simulink library "lib_transmission2"  (Simulink 4.1.1)
values from neighbouring files (symbols this model uses):
  logFlag = 1    [advSACompMaskInit.m]    (also in advSACompMaskInitR13.m)
undefined symbols (not defined in the file or in its folder): cyc_mph, fc_map_spd, fc_max_trq, fc_spd_scale, fc_trq_scale, fd_inertia, fd_loss, fd_ratio, gb_dnshift_load, gb_dnshift_spd, gb_gear_number_lookup, gb_gears_num, gb_inertia, gb_loss_const, gb_loss_input_spd_coeff, gb_loss_input_trq_coeff, gb_loss_output_spd_coeff, gb_loss_output_trq_coeff, gb_map_spd_out, gb_map_trq_in, gb_map_trq_out, gb_num_init, gb_ratio, gb_shift_delay, gb_spd_scale, gb_trq_scale, gb_upshift_load, gb_upshift_spd, htc_inertia, htc_k_adv, htc_k_adv_coast, htc_lockup, htc_lockup_load, htc_lockup_spd, htc_lu_gear_range, htc_max_coast_tr, htc_min_coast_tr, htc_pump_loss_spd, htc_pump_loss_trq_lockup, htc_pump_loss_trq_unlock, htc_sr, htc_sr_coast, htc_tr, htc_tr_coast, htc_unlock_spd, mc_map_spd, mc_max_trq, mc_overtrq_factor, mc_spd_scale, mc_trq_scale, tc_loss, tc_mc_to_fc_ratio, tx_eff_map, tx_map_spd, tx_map_trq, tx_pg_r, tx_pg_s, tx_speed_dep, vc_clutch_bool, vc_idle_spd ... (+2)
libraries: lib_controls x1, lib_etc x1, lib_controls2 x1, lib_transmission x1
(part 1 of 17)
settings Model: LastModifiedBy=mokeefe
settings Model: ModifiedComment=|
  | tmarkel -- Fri Sep 20 16:05:52 2002 -- Version 1.102
  | modified Pout/Pin calc block - moved !=0 check to before bombproof block; value after bombproof is never zero
  | 
  | there are still some issues with this calculation to be resolved at a later date
settings Model: ModifiedHistory=|
  | tmarkel -- Fri Sep 20 16:05:52 2002 -- Version 1.102
  | modified Pout/Pin calc block - moved !=0 check to before bombproof block; value after bombproof is never zero
  | 
  | there are still some issues with this calculation to be resolved at a later date
  | 
  | 
  | tmarkel -- Fri Sep 20 16:05:52 2002 -- Version 1.102
  | modified Pout/Pin calc block - moved !=0 check to before bombproof block; value after bombproof is never zero
  | 
  | there are still some issues with this calculation to be resolved at a later date
  | 
  | 
  | tmarkel -- Fri Sep 20 14:16:55 2002 -- Version 1.101
  | changed t loss when tx_eff=0 to be the total torque in request
  | 
  | abrooker -- Fri May 24 14:07:33 2002 -- Version 1.100
  | 
  | mokeefe -- Thu Apr 18 08:38:43 2002 -- Version 1.99
  | saving the model:
  | o "without the model browser open"
  | o with only top-level screen visible
  | o with "fit to view" enabled
  | o with "status bar" off and "toolbar" off
  | o with "prompt to update model history with each save" on

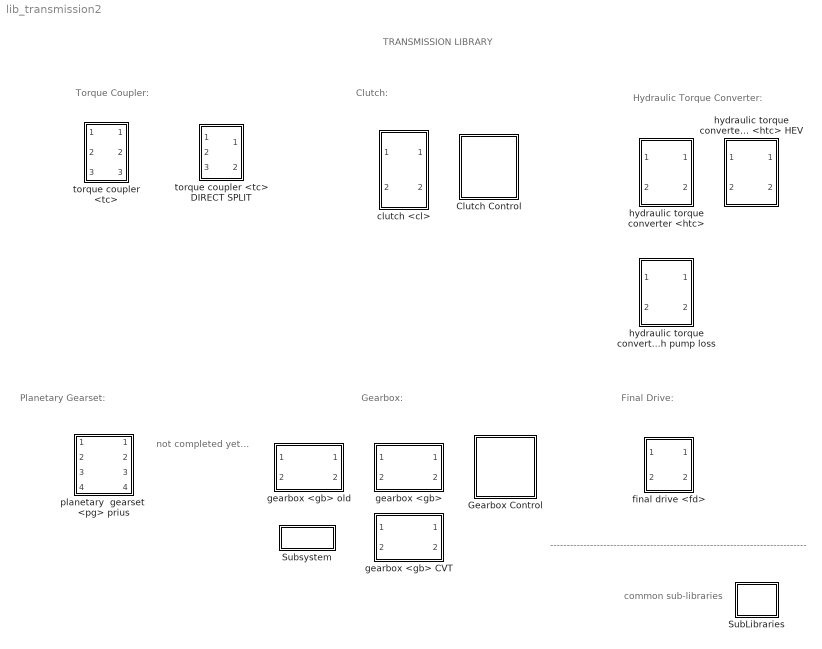
== system lib_transmission2 ==
  note: Torque Coupler:
  note: -----------------------------------------------------------------------------
  note: common
      | sub-libraries
  note: Clutch:
  note: Gearbox:
  note: Final Drive:
  note: Hydraulic Torque Converter:
  note: Planetary Gearset:
  note: not completed yet...
  note: TRANSMISSION LIBRARY
  Clutch Control : Subsystem
      settings: RTWFcnNameOpts=Auto  RTWFileNameOpts=Auto
  Gearbox Control : Subsystem
      settings: RTWFcnNameOpts=Auto  RTWFileNameOpts=Auto
  SubLibraries : Subsystem
      settings: RTWFcnNameOpts=Auto  RTWFileNameOpts=Auto
  Subsystem : Subsystem
      settings: RTWFcnNameOpts=Auto  RTWFileNameOpts=Auto
      mask Display: disp('GB Notes')
  clutch <cl> : Subsystem  mask(Stand-Alone Clutch Mask){generalName='cl', logPick=Don't Log, initFileName={}, modCell={}, imgFileName='bdi_cl.jpg', slip_spd=vc_launch_spd, maxtrq=max(fc_max_trq)*fc_trq_scale, DEBUG=OFF}
      mask prompts: generalName "General Name of this Component [char--evaluated]"; logPick "Log Variables to Workspace?"; initFileName "Initialization File(s) [cell array of char]"; modCell "Modification Cell [2 column cell array of param and val]"; imgFileName "Icon image file name [char--evaluated]"; slip_spd "Input shaft speed when clutch slips (rad/s):"; maxtrq "Maximum torque clutch can transmit:"
      mask help: Clutch for use with ADVISOR 2
      mask init:
      | % initialization via m-file script
      | advSACompMaskInit;
      settings: RTWFcnNameOpts=Auto  RTWFileNameOpts=Auto
      mask Help:
      | First input is req'd clutch output torque and speed, muxed together.
      | Second input is clutch state, with 1 => disengaged, 2 => slipping, and 3=> engaged.
      | Third input is available clutch input torque and limited clutch input speed.
      | First output is req'd clutch input torque and speed, muxed together.
      | Second output is available clutch output torque and limited clutch output speed.
      | The logic implemented by this block is as follows:
      |           IF (clutch is disengaged) THEN (req'd input torque=0), (req'd input speed=req'd output speed (the engine control is responsible for computing correct engine spin-down speed)), (avail. output torque=0), (limited output speed=req'd output speed)
      |           IF (clutch is slipping) THEN (req'd input torque=req'd output torque), (req'd input speed=user-defined slip speed), (avail. output torque=avail. input torque), (limited output speed=req'd output speed)
      |           IF (clutch is engaged) THEN (req'd input torque=req'd output torque), (req'd input speed=req'd output speed), (avail. output torque=avail. input torque), (limited output speed=limited input speed)
      | 
      | The clutch will transmit no more than its maximum torque as driving or braking torque.
      mask StyleString: edit,popup(Don't Log|Log),edit,edit,edit,edit,edit,popup(ON|OFF)
      mask Display: image(imread(imgFileName))
  final drive <fd> : Subsystem  mask(Stand-Alone Final Drive Mask){generalName='fd', logPick=Log, initFileName={}, modCell={}, imgFileName='bdi_fd.jpg', DEBUG=OFF}
      mask prompts: generalName "General Name of this Component [char]"; logPick "Log Variables to Workspace?"; initFileName "Initialization File(s) [cell array of char]"; modCell "Modification Cell [2 column cell array of param and val]"; imgFileName "Icon image file name [char--evaluated]"
      mask init:
      | % initialization via m-file script
      | advSACompMaskInit;
      settings: RTWFcnNameOpts=Auto  RTWFileNameOpts=Auto
      mask StyleString: edit,popup(Don't Log|Log),edit,edit,edit,popup(ON|OFF)
      mask Display: image(imread(imgFileName))
  gearbox <gb> : Subsystem  mask(Stand-Alone Gearbox Mask){generalName='gb', logPick=Log, initFileName={}, modCell={}, imgFileName='bdi_gb.jpg', DEBUG=OFF}
      mask prompts: generalName "General Name of this Component [char]"; logPick "Log Variables to Workspace?"; initFileName "Initialization File(s) [cell array of char]"; modCell "Modification Cell [2 column cell array of param and val]"; imgFileName "Icon image file name [char--evaluated]"
      mask init:
      | % initialization via m-file script
      | advSACompMaskInit;
      settings: RTWFcnNameOpts=Auto  RTWFileNameOpts=Auto
      mask StyleString: edit,popup(Don't Log|Log),edit,edit,edit,popup(ON|OFF)
      mask Display: image(imread(imgFileName))
  gearbox <gb> CVT : Subsystem  mask(Stand-Alone Gearbox Mask){generalName='gb', logPick=Log, initFileName={}, modCell={}, imgFileName='bdi_gb.jpg', DEBUG=OFF}
      mask prompts: generalName "General Name of this Component [char]"; logPick "Log Variables to Workspace?"; initFileName "Initialization File(s) [cell array of char]"; modCell "Modification Cell [2 column cell array of param and val]"; imgFileName "Icon image file name [char--evaluated]"
      mask init:
      | % initialization via m-file script
      | advSACompMaskInit;
      settings: RTWFcnNameOpts=Auto  RTWFileNameOpts=Auto
      mask StyleString: edit,popup(Don't Log|Log),edit,edit,edit,popup(ON|OFF)
      mask Display: image(imread(imgFileName))
  gearbox <gb> old : Subsystem  mask(Stand-Alone Gearbox Mask){generalName='gb', logPick=Log, initFileName={}, modCell={}, imgFileName='bdi_gb.jpg', DEBUG=OFF}
      mask prompts: generalName "General Name of this Component [char]"; logPick "Log Variables to Workspace?"; initFileName "Initialization File(s) [cell array of char]"; modCell "Modification Cell [2 column cell array of param and val]"; imgFileName "Icon image file name [char--evaluated]"
      mask init:
      | % initialization via m-file script
      | advSACompMaskInit;
      settings: RTWFcnNameOpts=Auto  RTWFileNameOpts=Auto
      mask StyleString: edit,popup(Don't Log|Log),edit,edit,edit,popup(ON|OFF)
      mask Display: image(imread(imgFileName))
  hydraulic torque converter <htc> : Subsystem  mask(Stand-Alone HTC Mask){generalName='htc', logPick=Log, initFileName={}, modCell={}, imgFileName='bdi_htc.jpg', DEBUG=OFF}
      mask prompts: generalName "General Name of this Component [char]"; logPick "Log Variables to Workspace?"; initFileName "Initialization File(s) [cell array of char]"; modCell "Modification Cell [2 column cell array of param and val]"; imgFileName "Icon image file name [char--evaluated]"
      mask init:
      | % initialization via m-file script
      | advSACompMaskInit;
      settings: RTWFcnNameOpts=Auto  RTWFileNameOpts=Auto
      mask StyleString: edit,popup(Don't Log|Log),edit,edit,edit,popup(ON|OFF)
      mask Display: image(imread(imgFileName))
  hydraulic torque converter <htc> HEV : Subsystem  mask(Stand-Alone HTC Mask){generalName='htc', logPick=Log, initFileName={}, modCell={}, imgFileName='bdi_htc.jpg', DEBUG=OFF}
      mask prompts: generalName "General Name of this Component [char]"; logPick "Log Variables to Workspace?"; initFileName "Initialization File(s) [cell array of char]"; modCell "Modification Cell [2 column cell array of param and val]"; imgFileName "Icon image file name [char--evaluated]"
      mask init:
      | % initialization via m-file script
      | advSACompMaskInit;
      settings: RTWFcnNameOpts=Auto  RTWFileNameOpts=Auto
      mask StyleString: edit,popup(Don't Log|Log),edit,edit,edit,popup(ON|OFF)
      mask Display: image(imread(imgFileName))
  hydraulic torque converter <htc> with pump loss : Subsystem  mask(Stand-Alone HTC Mask){generalName='htc', logPick=Log, initFileName={}, modCell={}, imgFileName='bdi_htc.jpg', DEBUG=OFF}
      mask prompts: generalName "General Name of this Component [char]"; logPick "Log Variables to Workspace?"; initFileName "Initialization File(s) [cell array of char]"; modCell "Modification Cell [2 column cell array of param and val]"; imgFileName "Icon image file name [char--evaluated]"
      mask init:
      | % initialization via m-file script
      | advSACompMaskInit;
      settings: RTWFcnNameOpts=Auto  RTWFileNameOpts=Auto
      mask StyleString: edit,popup(Don't Log|Log),edit,edit,edit,popup(ON|OFF)
      mask Display: image(imread(imgFileName))
  planetary  gearset  <pg> prius : Subsystem
      settings: RTWFcnNameOpts=Auto  RTWFileNameOpts=Auto
      mask Display: image(imread('bdi_psplit.jpg'))
  torque coupler <tc> : Subsystem  mask(Stand-Alone Torque Coupler Mask){generalName='tc', logPick=Don't Log, initFileName={}, modCell={}, imgFileName='bdi_tc.jpg', DEBUG=OFF}
      mask prompts: generalName "General Name of this Component [char--evaluated]"; logPick "Log Variables to Workspace?"; initFileName "Initialization File(s) [cell array of char]"; modCell "Modification Cell [2 column cell array of param and val]"; imgFileName "Icon image file name [char--evaluated]"
      mask init:
      | % initialization via m-file script
      | advSACompMaskInit;
      settings: RTWFcnNameOpts=Auto  RTWFileNameOpts=Auto
      mask StyleString: edit,popup(Don't Log|Log),edit,edit,edit,popup(ON|OFF)
      mask Display: image(imread(imgFileName))
  torque coupler <tc> DIRECT SPLIT : Subsystem  mask(Stand-Alone Direct Split Torque Coupler Mask){generalName='tc', logPick=Log, initFileName={}, modCell={}, imgFileName='bdi_tc.jpg', DEBUG=OFF}
      mask prompts: generalName "General Name of this Component [char--evaluated]"; logPick "Log Variables to Workspace?"; initFileName "Initialization File(s) [cell array of char]"; modCell "Modification Cell [2 column cell array of param and val]"; imgFileName "Icon image file name [char--evaluated]"
      mask init:
      | % initialization via m-file script
      | advSACompMaskInit;
      settings: RTWFcnNameOpts=Auto  RTWFileNameOpts=Auto
      mask StyleString: edit,popup(Don't Log|Log),edit,edit,edit,popup(ON|OFF)
      mask Display: image(imread(imgFileName))

== system lib_transmission2/Clutch Control ==
  Clutch Control : Subsystem
      settings: RTWFcnNameOpts=Auto  RTWFileNameOpts=Auto

== system lib_transmission2/Gearbox Control ==
  Gearbox Control manual shift logic : Subsystem
      settings: RTWFcnNameOpts=Auto  RTWFileNameOpts=Auto
  automatic transmission gearbox and htc advanced lock-up logic for htc shift logic for gearbox : Subsystem
      settings: RTWFcnNameOpts=Auto  RTWFileNameOpts=Auto
  automatic transmission gearbox and htc standard lockup logic for htc shift logic for gearbox : Subsystem
      settings: RTWFcnNameOpts=Auto  RTWFileNameOpts=Auto
  time lookup shift logic for gearbox : Subsystem
      settings: RTWFcnNameOpts=Auto  RTWFileNameOpts=Auto
  vehicle speed dependent shift logic for gearbox : Subsystem
      settings: RTWFcnNameOpts=Auto  RTWFileNameOpts=Auto

== system lib_transmission2/SubLibraries ==
  note: Trq and Spd at Output
      | (Nm) and (rad/s)
  note: Gear Ratio
      | (input spd/output spd)
  note: Trq loss
      | at input (Nm)
  note: gear ratio
      | (input/output spd)
  note: gear (1st, 2nd, etc.)
  note: data needs:
      | gb_ratio
  note: Below is the loss block for a gear box based
      | on loss equation--used with ADVISOR v. 3.1 and below
  note: X_lookup
  note: Y_lookup
  note: Z_discrete value
  note: looked up value
  note: X_lookup
  note: Y_lookup
  note: Z_discrete value
  note: looked up value
  3D discrete lookup table : Subsystem  mask{tx_map_spd=tx_map_spd, tx_map_trq=tx_map_trq, tx_eff_map=tx_eff_map}
      mask prompts: tx_map_spd "Row Lookup"; tx_map_trq "Column Lookup"; tx_eff_map "Lookup Matrix"
      settings: RTWFcnNameOpts=Auto  RTWFileNameOpts=Auto
  3D discrete lookup table (sfun) : Subsystem  mask{tx_map_spd=tx_map_spd, tx_map_trq=tx_map_trq, tx_eff_map=tx_eff_map}
      mask prompts: tx_map_spd "Row Lookup"; tx_map_trq "Column Lookup"; tx_eff_map "Lookup Matrix"
      settings: RTWFcnNameOpts=Auto  RTWFileNameOpts=Auto
  "gear determination (e.g., 1st gear, 2nd, etc.)" : Subsystem
      settings: RTWFcnNameOpts=Auto  RTWFileNameOpts=Auto
  loss (Nm) : Subsystem  mask{tx_eff_map=tx_eff_map, tx_map_trq=tx_map_trq, tx_map_spd=tx_map_spd, gb_spd_scale=gb_spd_scale, gb_trq_scale=gb_trq_scale}
      mask prompts: tx_eff_map "table of efficiency values (spd rad/s, trq Nm)"; tx_map_trq "vector of output torque values for lookup table (Nm)"; tx_map_spd "vector of output speeds for lookup table (rad/s)"; gb_spd_scale "Speed scale for the transmission gear box"; gb_trq_scale "Torque scale for the transmission gear box"
      settings: RTWFcnNameOpts=Auto  RTWFileNameOpts=Auto
  loss (Nm) old methodology : Subsystem
      settings: RTWFcnNameOpts=Auto  RTWFileNameOpts=Auto
  notes on  3D discrete lookup table : Subsystem
      settings: RTWFcnNameOpts=Auto  RTWFileNameOpts=Auto
  notes on  loss (Nm) : Subsystem
      settings: RTWFcnNameOpts=Auto  RTWFileNameOpts=Auto

== system lib_transmission2/Subsystem ==
  note: The gearbox old
      | model uses transmission
      | efficiency referenced from
      | the transmission output.
      |
      | The new file references from
      | the input.

== system lib_transmission2/clutch <cl> ==
  note: Clutch
      | Interface
  T & w output requested : Inport  Port=1  LatchInput=off
  T & w input achieved : Inport  Port=2  LatchInput=off
  clutch model and interface : Subsystem
      settings: RTWFcnNameOpts=Auto  RTWFileNameOpts=Auto
  T & w input request : Outport  Port=1
  T & w output achieved : Outport  Port=2
  tag scope: clReqOut=global, clSensors=global
  wires:
  T & w output requested/1 -> clutch model and interface/1(T & w output requested)
  clutch model and interface/2(Out1) -> T & w input request/1
  T & w input achieved/1 -> clutch model and interface/2(T & w input achieved)
  clutch model and interface/3(Out2) -> T & w output achieved/1
  clutch model and interface/4(sensors) -> [clSensors]
  clutch model and interface/1(required out) -> [clReqOut]
  [clControl] -> clutch model and interface/3(control)

== system lib_transmission2/final drive <fd> ==
  "torque and speed req'd at output side of final drive (Nm), (rad/s)" : Inport  Port=1  LatchInput=off
  "torque and speed avail. at input side of final drive (Nm), (rad/s)" : Inport  Port=2  LatchInput=off
  Block NOTES : Subsystem
      settings: RTWFcnNameOpts=Auto  RTWFileNameOpts=Auto
      mask Display: disp('Block\nNOTES')
  help : Subsystem
      settings: OpenFcn=web(['file:\\\' which('wheel_axle.htm')]);  RTWFcnNameOpts=Auto  RTWFileNameOpts=Auto
      mask Display: image(imread('doc_man.jpg'))
  model&interface : Subsystem
      settings: RTWFcnNameOpts=Auto  RTWFileNameOpts=Auto
  "torque and speed req'd at input side of final drive (Nm), (rad/s)" : Outport  Port=1  InitialOutput=0
  "torque and speed avail. at output side of final drive (Nm), (rad/s)" : Outport  Port=2  InitialOutput=0
  tag scope: fdReqOut=global, fdSensors=global
  wires:
  model&interface/1(out request) -> [fdReqOut]
  [fdControl] -> model&interface/3(control)
  model&interface/4(sensors) -> [fdSensors]
  "torque and speed req'd at output side of final drive (Nm), (rad/s)"/1 -> model&interface/1(T & w output request)
  "torque and speed avail. at input side of final drive (Nm), (rad/s)"/1 -> model&interface/2(T & w input achieved)
  model&interface/2(T & w input request) -> "torque and speed req'd at input side of final drive (Nm), (rad/s)"/1
  model&interface/3(T & w output achieved) -> "torque and speed avail. at output side of final drive (Nm), (rad/s)"/1

== system lib_transmission2/gearbox <gb> ==
  note: Gearbox
  "torque and speed req'd at output side of gearbox (Nm), (rad/s)" : Inport  Port=1  LatchInput=off
  "torque and speed avail. at input side of gearbox (Nm), (rad/s)" : Inport  Port=2  LatchInput=off
  Block NOTES : Subsystem
      settings: RTWFcnNameOpts=Auto  RTWFileNameOpts=Auto
      mask Display: disp('Block\nNOTES')
  gearbox model & interface : Subsystem
      settings: RTWFcnNameOpts=Auto  RTWFileNameOpts=Auto
  help : Subsystem
      settings: OpenFcn=web(['file:\\\' which('gearbox.htm')]);  RTWFcnNameOpts=Auto  RTWFileNameOpts=Auto
      mask Display: image(imread('doc_man.jpg'))
  "torque and speed req'd at input side of gearbox (Nm), (rad/s)" : Outport  Port=1  InitialOutput=0
  "torque and speed avail. at output side of gearbox (Nm), (rad/s)" : Outport  Port=2  InitialOutput=0
  tag scope: gbReqOut=global, gbSensors=global
  wires:
  gearbox model & interface/1(requested output) -> [gbReqOut]
  gearbox model & interface/2(trq and spd input request) -> "torque and speed req'd at input side of gearbox (Nm), (rad/s)"/1
  "torque and speed req'd at output side of gearbox (Nm), (rad/s)"/1 -> gearbox model & interface/1(trq and spd output request)
  "torque and speed avail. at input side of gearbox (Nm), (rad/s)"/1 -> gearbox model & interface/2(trq and spd input achieved)
  gearbox model & interface/3(trq and spd output achieved) -> "torque and speed avail. at output side of gearbox (Nm), (rad/s)"/1
  [gbControl] -> gearbox model & interface/3(controls)
  gearbox model & interface/4(sensors) -> [gbSensors]

== system lib_transmission2/gearbox <gb> CVT ==
  note: Gearbox
  "torque and speed req'd at output side of gearbox (Nm), (rad/s)" : Inport  Port=1  LatchInput=off
  "torque and speed avail. at input side of gearbox (Nm), (rad/s)" : Inport  Port=2  LatchInput=off
  Block NOTES : Subsystem
      settings: RTWFcnNameOpts=Auto  RTWFileNameOpts=Auto
      mask Display: disp('Block\nNOTES')
  CVT model & interface : Subsystem
      settings: RTWFcnNameOpts=Auto  RTWFileNameOpts=Auto
  help : Subsystem
      settings: OpenFcn=web(['file:\\\' which('gearbox.htm')]);  RTWFcnNameOpts=Auto  RTWFileNameOpts=Auto
      mask Display: image(imread('doc_man.jpg'))
  "torque and speed req'd at input side of gearbox (Nm), (rad/s)" : Outport  Port=1  InitialOutput=0
  "torque and speed avail. at output side of gearbox (Nm), (rad/s)" : Outport  Port=2  InitialOutput=0
  tag scope: gbReqOut=global, gbSensors=global
  wires:
  CVT model & interface/1(requested output) -> [gbReqOut]
  CVT model & interface/2(trq and spd input request) -> "torque and speed req'd at input side of gearbox (Nm), (rad/s)"/1
  "torque and speed req'd at output side of gearbox (Nm), (rad/s)"/1 -> CVT model & interface/1(trq and spd output request)
  "torque and speed avail. at input side of gearbox (Nm), (rad/s)"/1 -> CVT model & interface/2(trq and spd input achieved)
  CVT model & interface/3(trq and spd output achieved) -> "torque and speed avail. at output side of gearbox (Nm), (rad/s)"/1
  [gbControl] -> CVT model & interface/3(controls)
  CVT model & interface/4(sensors) -> [gbSensors]

== system lib_transmission2/gearbox <gb> old ==
  note: Gearbox
  "torque and speed req'd at output side of gearbox (Nm), (rad/s)" : Inport  Port=1  LatchInput=off
  "torque and speed avail. at input side of gearbox (Nm), (rad/s)" : Inport  Port=2  LatchInput=off
  Block NOTES : Subsystem
      settings: RTWFcnNameOpts=Auto  RTWFileNameOpts=Auto
      mask Display: disp('Block\nNOTES')
  gearbox model & interface : Subsystem
      settings: RTWFcnNameOpts=Auto  RTWFileNameOpts=Auto
  help : Subsystem
      settings: OpenFcn=web(['file:\\\' which('gearbox.htm')]);  RTWFcnNameOpts=Auto  RTWFileNameOpts=Auto
      mask Display: image(imread('doc_man.jpg'))
  "torque and speed req'd at input side of gearbox (Nm), (rad/s)" : Outport  Port=1  InitialOutput=0
  "torque and speed avail. at output side of gearbox (Nm), (rad/s)" : Outport  Port=2  InitialOutput=0
  tag scope: gbReqOut=global, gbSensors=global
  wires:
  gearbox model & interface/1(requested output) -> [gbReqOut]
  gearbox model & interface/2(trq and spd input request) -> "torque and speed req'd at input side of gearbox (Nm), (rad/s)"/1
  "torque and speed req'd at output side of gearbox (Nm), (rad/s)"/1 -> gearbox model & interface/1(trq and spd output request)
  "torque and speed avail. at input side of gearbox (Nm), (rad/s)"/1 -> gearbox model & interface/2(trq and spd input achieved)
  gearbox model & interface/3(trq and spd output achieved) -> "torque and speed avail. at output side of gearbox (Nm), (rad/s)"/1
  [gbControl] -> gearbox model & interface/3(controls)
  gearbox model & interface/4(sensors) -> [gbSensors]

== system lib_transmission2/hydraulic torque converter <htc> ==
  note: Hydraulic Torque Converter
  T & w output requested : Inport  Port=1  LatchInput=off
  T & w input available : Inport  Port=2  LatchInput=off
  conventional HTC  and Interface : Subsystem
      settings: RTWFcnNameOpts=Auto  RTWFileNameOpts=Auto
  T & w input requested : Outport  Port=1  InitialOutput=0
  T & w output available : Outport  Port=2  InitialOutput=0
  tag scope: htcReqOut=global, htcSensors=global
  wires:
  conventional HTC  and Interface/1(requested output) -> [htcReqOut]
  conventional HTC  and Interface/4(sensors) -> [htcSensors]
  conventional HTC  and Interface/2(trq and spd input request) -> T & w input requested/1
  conventional HTC  and Interface/3(trq and spd output achieved) -> T & w output available/1
  T & w output requested/1 -> conventional HTC  and Interface/1(trq and spd output request)
  T & w input available/1 -> conventional HTC  and Interface/2(trq and spd input achieved)
  [htcControl] -> conventional HTC  and Interface/3(control)

== system lib_transmission2/hydraulic torque converter <htc> HEV ==
  note: Hydraulic Torque Converter
  T & w output requested : Inport  Port=1  LatchInput=off
  T & w input available : Inport  Port=2  LatchInput=off
  HTC for parallel HEV and Interface : Subsystem
      settings: RTWFcnNameOpts=Auto  RTWFileNameOpts=Auto
  T & w input requested : Outport  Port=1  InitialOutput=0
  T & w output available : Outport  Port=2  InitialOutput=0
  tag scope: htcReqOut=global, htcSensors=global
  wires:
  HTC for parallel HEV and Interface/1(requested output) -> [htcReqOut]
  HTC for parallel HEV and Interface/4(sensors) -> [htcSensors]
  HTC for parallel HEV and Interface/2(trq and spd input request) -> T & w input requested/1
  HTC for parallel HEV and Interface/3(trq and spd output achieved) -> T & w output available/1
  T & w output requested/1 -> HTC for parallel HEV and Interface/1(trq and spd output request)
  T & w input available/1 -> HTC for parallel HEV and Interface/2(trq and spd input achieved)
  [htcControl] -> HTC for parallel HEV and Interface/3(control)

== system lib_transmission2/hydraulic torque converter <htc> with pump loss ==
  note: Hydraulic Torque Converter
  T & w output requested : Inport  Port=1  LatchInput=off
  T & w input available : Inport  Port=2  LatchInput=off
  conventional HTC  and Interface : Subsystem
      settings: RTWFcnNameOpts=Auto  RTWFileNameOpts=Auto
  T & w input requested : Outport  Port=1  InitialOutput=0
  T & w output available : Outport  Port=2  InitialOutput=0
  tag scope: htcReqOut=global, htcSensors=global
  wires:
  conventional HTC  and Interface/1(requested output) -> [htcReqOut]
  conventional HTC  and Interface/4(sensors) -> [htcSensors]
  conventional HTC  and Interface/2(trq and spd input request) -> T & w input requested/1
  conventional HTC  and Interface/3(trq and spd output achieved) -> T & w output available/1
  T & w output requested/1 -> conventional HTC  and Interface/1(trq and spd output request)
  T & w input available/1 -> conventional HTC  and Interface/2(trq and spd input achieved)
  [htcControl] -> conventional HTC  and Interface/3(control)

== system lib_transmission2/planetary  gearset  <pg> prius ==
  "torque and speed required from ring gear (Nm), (rad/s)1" : Inport  Port=1  LatchInput=off
  "torque and speed avail. from fuel converter (Nm), (rad/s)" : Inport  Port=2  LatchInput=off
  "torque and speed avail. from generator (Nm), (rad/s)" : Inport  Port=3  LatchInput=off
  "torque and speed available from motor (Nm), (rad/s)1" : Inport  Port=4  LatchInput=off
  Demux{,1..3} (4 alike) : Demux  Outputs=2  BusSelectionMode=off
  Mux{,1..3} (4 alike) : Mux  Inputs=2
      settings: DisplayOption=none
  Sum2 : Sum  Inputs=++  SaturateOnIntegerOverflow=on
  Sum5 : Sum  Inputs=+-  SaturateOnIntegerOverflow=on
  Sum6 : Sum  Inputs=+-  SaturateOnIntegerOverflow=on
  Terminator : Terminator
  Terminator2 : Terminator
  engine_to_generator : Gain  Gain=-tx_pg_s/(tx_pg_r+tx_pg_s)  Multiplication=Element-wise(K.*u)  SaturateOnIntegerOverflow=on
  gain : Gain  Gain=tx_pg_r/(tx_pg_r+tx_pg_s)  Multiplication=Element-wise(K.*u)  SaturateOnIntegerOverflow=on
  gain2 : Gain  Gain=1+tx_pg_r/tx_pg_s  Multiplication=Element-wise(K.*u)  SaturateOnIntegerOverflow=on
  gain5 : Gain  Gain=tx_pg_r/tx_pg_s  Multiplication=Element-wise(K.*u)  SaturateOnIntegerOverflow=on
  spd out : ToWorkspace  VariableName=pg_spd_out_r  SampleTime=0  SaveFormat=Array
      settings: MaxDataPoints=100000
  trq out : ToWorkspace  VariableName=pg_trq_out_r  SampleTime=0  SaveFormat=Array
      settings: MaxDataPoints=100000
  "torque and speed req'd from fuel converter (Nm), (rad/s)" : Outport  Port=1  InitialOutput=0
  "torque and speed req'd from generator (Nm), (rad/s)" : Outport  Port=2  InitialOutput=0
  "torque and speed req'd from motor (Nm), (rad/s)1" : Outport  Port=3  InitialOutput=0
  "torque and speed available to final drive (Nm), (rad/s)1" : Outport  Port=4  InitialOutput=0
  tag scope: pgs_trq_spd_r=global
  wires:
  "torque and speed available from motor (Nm), (rad/s)1"/1 -> Demux3/1
  Demux3/2 -> gain5/1, Mux3/2
  Demux3/1 -> Sum2/2
  Mux3/1 -> "torque and speed available to final drive (Nm), (rad/s)1"/1
  Sum2/1 -> Mux3/1
  Sum5/1 -> Mux1/2
  engine_to_generator/1 -> Mux1/1
  Mux1/1 -> "torque and speed req'd from generator (Nm), (rad/s)"/1
  Sum6/1 -> Mux2/1
  Mux2/1 -> "torque and speed req'd from motor (Nm), (rad/s)1"/1
  gain2/1 -> Sum5/1
  Demux/2 -> Terminator/1
  Demux/1 -> Terminator2/1
  "torque and speed avail. from generator (Nm), (rad/s)"/1 -> Demux/1
  Demux1/1 -> engine_to_generator/1, gain/1
  Demux1/2 -> gain2/1
  "torque and speed avail. from fuel converter (Nm), (rad/s)"/1 -> Demux1/1
  gain5/1 -> Sum5/2
  [fc_trq_req] -> Mux/1
  [fc_spd_req] -> Mux/2
  Mux/1 -> "torque and speed req'd from fuel converter (Nm), (rad/s)"/1
  Demux2/1 -> Sum6/1, trq out/1
  Demux2/2 -> Mux2/2, spd out/1
  gain/1 -> Sum2/1, Sum6/2
  "torque and speed required from ring gear (Nm), (rad/s)1"/1 -> [pgs_trq_spd_r], Demux2/1

== system lib_transmission2/torque coupler <tc> ==
  note: Torque Coupler
  "torque and speed req'd at output side of torque coupler (Nm), (rad/s)" : Inport  Port=1  LatchInput=off
  "torque and speed avail. at main input (Nm), (rad/s)" : Inport  Port=2  LatchInput=off
  "torque and speed avail. at motor input to tc (Nm), (rad/s)" : Inport  Port=3  LatchInput=off
  tc model & interface : Subsystem
      settings: RTWFcnNameOpts=Auto  RTWFileNameOpts=Auto
  "torque and speed req'd at main input to torque coupler (Nm), (rad/s)" : Outport  Port=1  InitialOutput=0
  "torque and speed req'd at motor input to torque coupler (Nm), (rad/s)" : Outport  Port=2  InitialOutput=0
  "torque and speed avail. at output side of torque coupler (Nm), (rad/s)" : Outport  Port=3  InitialOutput=0
  tag scope: tcReqOut=global, tcSensors=global
  wires:
  "torque and speed req'd at output side of torque coupler (Nm), (rad/s)"/1 -> tc model & interface/1(trq and spd output request)
  "torque and speed avail. at main input (Nm), (rad/s)"/1 -> tc model & interface/2(trq and spd avail. at main input)
  "torque and speed avail. at motor input to tc (Nm), (rad/s)"/1 -> tc model & interface/3(trq and spd avail. at motor input to tc)
  [tcControl] -> tc model & interface/4(controls)
  tc model & interface/1(requested output) -> [tcReqOut]
  tc model & interface/2(trq and spd req'd at main input) -> "torque and speed req'd at main input to torque coupler (Nm), (rad/s)"/1
  tc model & interface/3(trq and spd req'd at motor input to torque coupler) -> "torque and speed req'd at motor input to torque coupler (Nm), (rad/s)"/1
  tc model & interface/4(trq and spd avail. at output side of torque coupler) -> "torque and speed avail. at output side of torque coupler (Nm), (rad/s)"/1
  tc model & interface/5(sensors) -> [tcSensors]

== system lib_transmission2/torque coupler <tc> DIRECT SPLIT ==
  note: Torque Coupler
  "torque and speed req'd at output side of torque coupler (Nm), (rad/s)" : Inport  Port=1  LatchInput=off
  "torque and speed avail. at main input (Nm), (rad/s)" : Inport  Port=2  LatchInput=off
  "torque and speed avail. at motor input to tc (Nm), (rad/s)" : Inport  Port=3  LatchInput=off
  tc direct split model & interface : Subsystem
      settings: RTWFcnNameOpts=Auto  RTWFileNameOpts=Auto
  "torque and speed req'd at main input to torque coupler (Nm), (rad/s)" : Outport  Port=1  InitialOutput=0
  "torque and speed avail. at output side of torque coupler (Nm), (rad/s)" : Outport  Port=2  InitialOutput=0
  tag scope: tcReqOut=global, tcSensors=global
  wires:
  "torque and speed req'd at output side of torque coupler (Nm), (rad/s)"/1 -> tc direct split model & interface/1(trq and spd output request)
  "torque and speed avail. at main input (Nm), (rad/s)"/1 -> tc direct split model & interface/2(trq and spd avail. at main input)
  "torque and speed avail. at motor input to tc (Nm), (rad/s)"/1 -> tc direct split model & interface/3(trq and spd avail. at motor input to tc)
  [tcControl] -> tc direct split model & interface/4(control)
  tc direct split model & interface/1(required output) -> [tcReqOut]
  tc direct split model & interface/2(trq and spd req'd at main input) -> "torque and speed req'd at main input to torque coupler (Nm), (rad/s)"/1
  tc direct split model & interface/3(trq and spd avail. at output side of torque coupler) -> "torque and speed avail. at output side of torque coupler (Nm), (rad/s)"/1
  tc direct split model & interface/4(sensors) -> [tcSensors]

== system lib_transmission2/Clutch Control/Clutch Control ==
  Bus Creator : BusCreator  Inputs=3
  Bus Selector : BusSelector  OutputSignals=mpha  MuxedOutput=off
  Bus Selector1 : BusSelector  OutputSignals=shifting  MuxedOutput=off
  Bus Selector2 : BusSelector  OutputSignals=gb_spd_in_a  MuxedOutput=off
  Bus Selector3 : BusSelector  OutputSignals=clutch_trq_out_r  MuxedOutput=off
  Bus Selector4 : BusSelector  OutputSignals=clutch_spd_out_r  MuxedOutput=off
  Bus Selector5 : BusSelector  OutputSignals=veh_spd_a_rec  MuxedOutput=off
  Bus Selector6 : BusSelector  OutputSignals=cycle_mph_r  MuxedOutput=off
  Bus Selector7 : BusSelector  OutputSignals=v_ave_req  MuxedOutput=off
  Clutch Control : Subsystem  TreatAsAtomicUnit=on
      settings: RTWFcnNameOpts=Auto  RTWFileNameOpts=Auto
  Memory1 : Memory  X0=0  InheritSampleTime=off
      settings: RTWStateStorageClass=Auto
  Memory2 : Memory  X0=cyc_mph(1,2)  InheritSampleTime=off
      settings: RTWStateStorageClass=Auto
  Memory3 : Memory  X0=0  InheritSampleTime=off
      settings: RTWStateStorageClass=Auto
  Memory4 : Memory  X0=cyc_mph(1,2)  InheritSampleTime=off
      settings: RTWStateStorageClass=Auto
  tag scope: clControl=global
  wires:
  Memory4/1 -> Clutch Control/7(cyc_mph_r)
  Memory3/1 -> Clutch Control/6(veh_spd_a_rec)
  Memory2/1 -> Clutch Control/5(mpha)
  Memory1/1 -> Clutch Control/2(gb_spd_in_a)
  Clutch Control/3(launch_flag) -> Bus Creator/3  "launch_flag"
  Bus Selector4/1 -> Clutch Control/4(w_cl_out)  "<clutch_spd_out_r>"
  Bus Selector3/1 -> Clutch Control/3(T_cl_out)  "<clutch_trq_out_r>"
  [clReqOut] -> Bus Selector4/1, Bus Selector3/1
  Bus Selector2/1 -> Memory1/1  "<gb_spd_in_a>"
  [gbSensors] -> Bus Selector2/1
  Bus Selector1/1 -> Clutch Control/1(shifting)  "<shifting>"
  [gbControl] -> Bus Selector1/1
  Clutch Control/2(launch_speed) -> Bus Creator/2  "launch_speed"
  Clutch Control/1(clutch_state) -> Bus Creator/1  "clutch_state"
  Bus Creator/1 -> [clControl]
  [vehSensors] -> Bus Selector/1
  Bus Selector/1 -> Memory2/1  "<mpha>"
  [vehSensors] -> Bus Selector5/1
  Bus Selector5/1 -> Memory3/1  "<veh_spd_a_rec>"
  [cycReqOut] -> Bus Selector6/1
  Bus Selector6/1 -> Memory4/1  "<cycle_mph_r>"
  [vehReqOut] -> Bus Selector7/1
  Bus Selector7/1 -> Clutch Control/8(v_ave_req)  "<v_ave_req>"

== system lib_transmission2/Gearbox Control/Gearbox Control manual shift logic ==
  Bus Selector : BusSelector  OutputSignals=acc_mech_trq_a  MuxedOutput=off
  Bus Selector1 : BusSelector  OutputSignals=mpha  MuxedOutput=off
  Bus Selector10 : BusSelector  OutputSignals=eta_gb  MuxedOutput=off
  Bus Selector2 : BusSelector  OutputSignals=cycle_mph_r  MuxedOutput=off
  Bus Selector3 : BusSelector  OutputSignals=veh_spd_a_rec  MuxedOutput=off
  Bus Selector4 : BusSelector  OutputSignals=slip_limited  MuxedOutput=off
  Bus Selector7 : BusSelector  OutputSignals=gb_trq_out_r  MuxedOutput=off
  Bus Selector8 : BusSelector  OutputSignals=gb_spd_out_r  MuxedOutput=off
  Bus Selector9 : BusSelector  OutputSignals=gb_spd_in_a  MuxedOutput=off
  Memory{,1,3,5} (4 alike) : Memory  X0=0  InheritSampleTime=off
      settings: RTWStateStorageClass=Auto
  Memory2 : Memory  X0=cyc_mph(1,2)  InheritSampleTime=off
      settings: RTWStateStorageClass=Auto
  Memory4 : Memory  X0=cyc_mph(1,2)  InheritSampleTime=off
      settings: RTWStateStorageClass=Auto
  Mux1 : Mux  Inputs=3
  manual shift logic : Subsystem  TreatAsAtomicUnit=on
      settings: RTWFcnNameOpts=Auto  RTWFileNameOpts=Auto
  tag scope: gbControl=global
  wires:
  Memory4/1 -> manual shift logic/7("cyc_mph_r, t=(i-1)")
  Memory3/1 -> manual shift logic/8("veh_spd_a_rec, t=(i-1)")
  Memory2/1 -> manual shift logic/6("mpha, t=(i-1)")
  Memory1/1 -> manual shift logic/2("gb_spd_in_a, t=(i-1)")
  Memory/1 -> manual shift logic/1("eta_gb, t=(i-1)")
  [gbReqOut] -> Bus Selector7/1, Bus Selector8/1
  Bus Selector7/1 -> manual shift logic/4(T_gb_out)  "<gb_trq_out_r>"
  Bus Selector8/1 -> manual shift logic/3(w_gb_out)  "<gb_spd_out_r>"
  Bus Selector9/1 -> Memory1/1  "<gb_spd_in_a>"
  Bus Selector10/1 -> Memory/1  "<eta_gb>"
  [gbSensors] -> Bus Selector9/1, Bus Selector10/1
  Mux1/1 -> [gbControl]
  manual shift logic/3(gear number) -> Mux1/3  "gear_number"
  manual shift logic/2(shifting) -> Mux1/2  "shifting"
  manual shift logic/1(gear ratio) -> Mux1/1  "gear_ratio"
  [accSensors] -> Bus Selector/1
  Bus Selector/1 -> Memory5/1  "<acc_mech_trq_a>"
  Memory5/1 -> manual shift logic/5(acc_mech_trq_est)
  [vehSensors] -> Bus Selector1/1
  Bus Selector1/1 -> Memory2/1  "<mpha>"
  [cycReqOut] -> Bus Selector2/1
  Bus Selector2/1 -> Memory4/1  "<cycle_mph_r>"
  [vehSensors] -> Bus Selector3/1
  Bus Selector3/1 -> Memory3/1  "<veh_spd_a_rec>"
  [vehReqOut] -> Bus Selector4/1
  Bus Selector4/1 -> manual shift logic/9(slip_limited)  "<slip_limited>"

== system lib_transmission2/Gearbox Control/automatic transmission gearbox and htc advanced lock-up logic for htc shift logic for gearbox ==
  gearbox controls : Inport  Port=1  LatchInput=off
  htc control : Inport  Port=2  LatchInput=off
  Demux : Demux  Outputs=2  BusSelectionMode=off
  Demux2 : Demux  Outputs=3  BusSelectionMode=off
  Goto Tag Visibility : GotoTagVisibility  GotoTag=gear_number
  Goto Tag Visibility1 : GotoTagVisibility  GotoTag=shifting
  Goto Tag Visibility2 : GotoTagVisibility  GotoTag=gear_ratio
  Goto Tag Visibility3 : GotoTagVisibility  GotoTag=shifting
  Goto Tag Visibility4 : GotoTagVisibility  GotoTag=locked_up
  gearbox control for use w/ AT : Subsystem
      settings: RTWFcnNameOpts=Auto  RTWFileNameOpts=Auto
  tag scope: gear_number=global, gear_number=scoped, gear_ratio=global, gear_ratio=scoped, locked_up=global, locked_up=scoped, shifting=global, shifting=scoped
  wires:
  gearbox control for use w/ AT/3("shifting, out") -> [shifting]
  [w_gb_out] -> gearbox control for use w/ AT/3(gb_spd_out_r)
  [T_gb_out] -> gearbox control for use w/ AT/2(gb_trq_out_r)
  [slip_limited] -> gearbox control for use w/ AT/4(tires are at traction limit)
  [eta_gb] -> gearbox control for use w/ AT/1(eta_gb)
  gearbox control for use w/ AT/1("gear number, out") -> [gear_number]
  gearbox control for use w/ AT/2("gear ratio, out") -> [gear_ratio]
  gearbox control for use w/ AT/4(locked up) -> [locked_up]
  gearbox controls/1 -> Demux2/1
  Demux2/1 -> [gear_ratio]
  Demux2/2 -> [shifting]
  Demux2/3 -> [gear_number]
  htc control/1 -> Demux/1
  Demux/1 -> [shifting]
  Demux/2 -> [locked_up]

== system lib_transmission2/Gearbox Control/automatic transmission gearbox and htc standard lockup logic for htc shift logic for gearbox ==
  eta_gb(t-1) : Inport  Port=1  LatchInput=off
  T_gb_out (request)(t) : Inport  Port=2  LatchInput=off
  w_gb_out (request)(t) : Inport  Port=3  LatchInput=off
  Bus Creator : BusCreator  Inputs=3
  Bus Creator1 : BusCreator  Inputs=2
  Goto Tag Visibility : GotoTagVisibility  GotoTag=acc_mech_trq_est
  Goto Tag Visibility1 : GotoTagVisibility  GotoTag=locked_up_last
  gearbox control for use w/ AT : Subsystem
      settings: RTWFcnNameOpts=Auto  RTWFileNameOpts=Auto
  tag scope: acc_mech_trq_est=scoped, locked_up_last=scoped
  wires:
  gearbox control for use w/ AT/4(locked up) -> [locked_up]
  gearbox control for use w/ AT/2("gear ratio, out") -> [gear_ratio]
  gearbox control for use w/ AT/1("gear number, out") -> [gear_number]
  [eta_gb_last] -> gearbox control for use w/ AT/1(eta_gb)
  [slip_limited] -> gearbox control for use w/ AT/4(tires are at traction limit)
  [T_gb_out] -> gearbox control for use w/ AT/2(gb_trq_out_r)
  [w_gb_out] -> gearbox control for use w/ AT/3(gb_spd_out_r)
  gearbox control for use w/ AT/3("shifting, out") -> [shifting]
  [gear_ratio] -> Bus Creator/1  "gear_ratio"
  [shifting] -> Bus Creator/2  "shifting"
  [gear_number] -> Bus Creator/3  "gear_number"
  [shifting] -> Bus Creator1/1  "shifting"
  [locked_up] -> Bus Creator1/2  "locked_up"
  eta_gb(t-1)/1 -> [eta_gb_last]
  T_gb_out (request)(t)/1 -> [T_gb_out]
  w_gb_out (request)(t)/1 -> [w_gb_out]

== system lib_transmission2/Gearbox Control/time lookup shift logic for gearbox ==
  Bus Selector11 : BusSelector  OutputSignals=signal2  MuxedOutput=off
  Mux2 : Mux  Inputs=3
  lookup : Subsystem
      settings: RTWFcnNameOpts=Auto  RTWFileNameOpts=Auto
  tag scope: gbControl=global
  wires:
  lookup/1(gear ratio) -> Mux2/1
  lookup/2(shifting) -> Mux2/2
  lookup/3(gear number) -> Mux2/3
  Mux2/1 -> [gbControl]
  [whSensors] -> Bus Selector11/1
  Bus Selector11/1 -> lookup/1(time)  "<signal2>"

== system lib_transmission2/Gearbox Control/vehicle speed dependent shift logic for gearbox ==
  Bus Selector : BusSelector  OutputSignals=signal2  MuxedOutput=off
  Mux : Mux  Inputs=3
  speed dependent : Subsystem
      settings: RTWFcnNameOpts=Auto  RTWFileNameOpts=Auto
  tag scope: gbControl=global
  wires:
  speed dependent/1(gear ratio) -> Mux/1
  speed dependent/2(shifting) -> Mux/2
  speed dependent/3(gear number) -> Mux/3
  Mux/1 -> [gbControl]
  [whSensors] -> Bus Selector/1
  Bus Selector/1 -> speed dependent/1(v_req_limited)  "<signal2>"

== system lib_transmission2/SubLibraries/3D discrete lookup table ==
  lookup speed (rad/s) : Inport  Port=1  LatchInput=off
  lookup trq (Nm) : Inport  Port=2  LatchInput=off
  "gear_number  (e.g., 1, 2, 3)" : Inport  Port=3  LatchInput=off
  Mux : Mux  Inputs=3
  Saturation : Saturate  UpperLimit=max(tx_map_spd)  LowerLimit=min(tx_map_spd)  LinearizeAsGain=on
  Saturation1 : Saturate  UpperLimit=max(tx_map_trq)  LowerLimit=min(tx_map_trq)  LinearizeAsGain=on
  Saturation2 : Saturate  UpperLimit=size(tx_eff_map,3)  LowerLimit=1  LinearizeAsGain=on
  interp2d : MATLABFcn  MATLABFcn=interp2(tx_map_trq, tx_map_spd, tx_eff_map(:,:,u(3)),u(2),u(1))  OutputDimensions=1  OutputSignalType=real  Output1D=on
  tx_eff : Outport  Port=1
  wires:
  Mux/1 -> interp2d/1
  interp2d/1 -> tx_eff/1
  lookup speed (rad/s)/1 -> Saturation/1
  Saturation/1 -> Mux/1
  lookup trq (Nm)/1 -> Saturation1/1
  Saturation1/1 -> Mux/2
  "gear_number  (e.g., 1, 2, 3)"/1 -> Saturation2/1
  Saturation2/1 -> Mux/3

== system lib_transmission2/SubLibraries/3D discrete lookup table (sfun) ==
  lookup speed (rad/s) : Inport  Port=1  LatchInput=off
  lookup trq (Nm) : Inport  Port=2  LatchInput=off
  "gear_number  (e.g., 1, 2, 3)" : Inport  Port=3  LatchInput=off
  Mux : Mux  Inputs=3
  Saturation : Saturate  UpperLimit=max(tx_map_spd)  LowerLimit=min(tx_map_spd)  LinearizeAsGain=on
  Saturation1 : Saturate  UpperLimit=max(tx_map_trq)  LowerLimit=min(tx_map_trq)  LinearizeAsGain=on
  Saturation2 : Saturate  UpperLimit=size(tx_eff_map,3)  LowerLimit=1  LinearizeAsGain=on
  discrete interp2d : S-Function  FunctionName=sfun_discreteLookup3d  Parameters=tx_map_trq, tx_map_spd, tx_eff_map  PortCounts=[]  SFunctionModules=''
  tx_eff : Outport  Port=1
  wires:
  Saturation2/1 -> Mux/3
  "gear_number  (e.g., 1, 2, 3)"/1 -> Saturation2/1
  Saturation1/1 -> Mux/2
  lookup trq (Nm)/1 -> Saturation1/1
  Saturation/1 -> Mux/1
  lookup speed (rad/s)/1 -> Saturation/1
  Mux/1 -> discrete interp2d/1
  discrete interp2d/1 -> tx_eff/1

== system lib_transmission2/SubLibraries/gear determination (e.g., 1st gear, 2nd, etc.) ==
  in_1 : Inport  Port=1  LatchInput=off
  Look-Up Table : Lookup  InputValues=fliplr([gb_ratio(1)+0.00001,gb_ratio(2:end)])  OutputValues=fliplr( [1:length(gb_ratio)] )
  Rounding Function : Rounding  Operator=round
  index of lower bounding map : Outport  Port=1  InitialOutput=0
  wires:
  in_1/1 -> Look-Up Table/1
  Look-Up Table/1 -> Rounding Function/1
  Rounding Function/1 -> index of lower bounding map/1

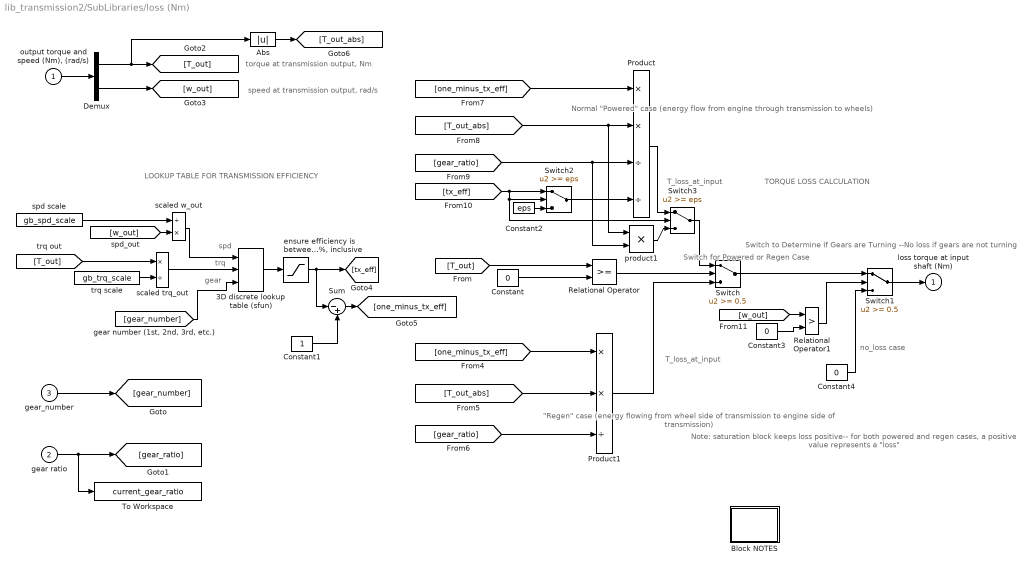
== system lib_transmission2/SubLibraries/loss (Nm) ==
  note: LOOKUP TABLE FOR TRANSMISSION EFFICIENCY
  note: T_loss_at_input
  note: "Regen" case
      | (energy flowing from
      | wheel side of transmission
      | to engine side of transmission)
  note: T_loss_at_input
  note: Normal "Powered" case
      | (energy flow from engine
      | through transmission to wheels)
  note: Switch to Determine
      | if Gears are Turning
      | --No loss if gears
      | are not turning
  note: Switch for Powered
      |  or Regen Case
  note: Note: saturation block keeps
      | loss positive-- for both powered
      | and regen cases, a
      | positive value represents a "loss"
  note: no_loss case
  note: speed at transmission output, rad/s
  note: torque at transmission output, Nm
  note: spd
  note: trq
  note: gear
  note: TORQUE LOSS CALCULATION
  "output torque and speed (Nm), (rad/s)" : Inport  Port=1  LatchInput=off
  gear ratio : Inport  Port=2  LatchInput=off
  gear_number : Inport  Port=3  LatchInput=off
  3D discrete lookup table (sfun) : lib_transmission/SubLibraries/3D discrete lookup table (sfun)  tx_map_spd=tx_map_spd  tx_map_trq=tx_map_trq  tx_eff_map=tx_eff_map
  Abs : Abs  SaturateOnIntegerOverflow=on
  Block NOTES : Subsystem
      settings: RTWFcnNameOpts=Auto  RTWFileNameOpts=Auto
      mask Display: disp('Block\nNOTES')
  Constant : Constant  Value=0
  Constant1 : Constant  Value=1
  Constant2 : Constant  Value=eps
  Constant3 : Constant  Value=0
  Constant4 : Constant  Value=0
  Demux : Demux  Outputs=2  BusSelectionMode=off
  Product : Product  Inputs=**//  Multiplication=Element-wise(.*)  SaturateOnIntegerOverflow=on
  Product1 : Product  Inputs=**/  Multiplication=Element-wise(.*)  SaturateOnIntegerOverflow=on
  Relational Operator : RelationalOperator  Operator=>=
  Relational Operator1 : RelationalOperator  Operator=>
  Sum : Sum  Inputs=|-+  SaturateOnIntegerOverflow=on
  Switch : Switch  Threshold=0.5
  Switch1 : Switch  Threshold=0.5
  Switch2 : Switch  Threshold=eps
  Switch3 : Switch  Threshold=eps
  To Workspace : ToWorkspace  VariableName=current_gear_ratio  SampleTime=-1  SaveFormat=Array
      settings: MaxDataPoints=1
  "ensure efficiency is between  0% and 100%, inclusive" : Saturate  UpperLimit=1  LowerLimit=0  LinearizeAsGain=on
  product1 : Product  Inputs=2  Multiplication=Element-wise(.*)  SaturateOnIntegerOverflow=on
  scaled trq_out : Product  Inputs=*/  Multiplication=Element-wise(.*)  SaturateOnIntegerOverflow=on
  scaled w_out : Product  Inputs=/*  Multiplication=Element-wise(.*)  SaturateOnIntegerOverflow=on
  spd scale : Constant  Value=gb_spd_scale
  trq scale : Constant  Value=gb_trq_scale
  loss torque at input shaft (Nm) : Outport  Port=1  InitialOutput=0
  wires:
  "output torque and speed (Nm), (rad/s)"/1 -> Demux/1
  Demux/2 -> [w_out]
  [gear_number] -> 3D discrete lookup table (sfun)/3
  Relational Operator/1 -> Switch/2
  Constant/1 -> Relational Operator/2
  [T_out] -> Relational Operator/1
  Product1/1 -> Switch/3
  [one_minus_tx_eff] -> Product1/1
  [gear_ratio] -> Product1/3
  [T_out_abs] -> Product1/2
  [one_minus_tx_eff] -> Product/1
  [T_out_abs] -> Product/2, product1/1
  [gear_ratio] -> Product/3, product1/2
  Switch1/1 -> loss torque at input shaft (Nm)/1
  Constant4/1 -> Switch1/3
  [w_out] -> Relational Operator1/1
  Constant3/1 -> Relational Operator1/2
  Relational Operator1/1 -> Switch1/2
  Demux/1 -> [T_out], Abs/1
  Abs/1 -> [T_out_abs]
  Switch/1 -> Switch1/1
  3D discrete lookup table (sfun)/1 -> "ensure efficiency is between  0% and 100%, inclusive"/1
  "ensure efficiency is between  0% and 100%, inclusive"/1 -> [tx_eff], Sum/1
  scaled w_out/1 -> 3D discrete lookup table (sfun)/1
  [T_out] -> scaled trq_out/1
  scaled trq_out/1 -> 3D discrete lookup table (sfun)/2
  trq scale/1 -> scaled trq_out/2
  Constant1/1 -> Sum/2
  Sum/1 -> [one_minus_tx_eff]
  [w_out] -> scaled w_out/2
  spd scale/1 -> scaled w_out/1
  gear ratio/1 -> [gear_ratio], To Workspace/1
  gear_number/1 -> [gear_number]
  Switch2/1 -> Product/4
  [tx_eff] -> Switch2/1, Switch2/2, Switch3/2
  Constant2/1 -> Switch2/3
  Switch3/1 -> Switch/1
  Product/1 -> Switch3/1
  product1/1 -> Switch3/3
